simulink model "busdemo"  (Simulink 7.6)
settings: Solver=VariableStepDiscrete  StartTime=0.0  StopTime=10  MaxStep=.05  RelTol=1e-3
libraries: simulink x2
Description:
  | Demonstration model for vector, matrix, and composite signals
  | 
  | This model introduces you to the following Simulink(R) concepts:
  | 
  |  * Distinguishing vector, matrix, and bus/composite signals
  |  * Understanding signal line formats
  |  * Displaying and understanding signal dimensions
  |  * Using the Bus Creator and the Bus Selector blocks
  |  * Viewing matrix signals on a Simulink Scope
  |  * Highlighting blocks in the Simulink diagram
settings Model: Creator=The MathWorks Inc.  CovMetricSettings=d  ExtModeTrigMode=oneshot  ExtModeArmWhenConnect=off  ExtModeAutoUpdateStatusClock=off
settings DataIOCC: LimitDataPoints=off  SaveOutput=off  SignalLogging=off  SaveTime=off
settings OptimizationCC: BlockReduction=off  BooleanDataType=off  InlineInvariantSignals=on  InitFltsAndDblsToZero=on  BufferReusableBoundary=off
settings DebuggingCC: SaveWithParameterizedLinksMsg=none  SignalResolutionControl=TryResolveAllWithWarning  SolverPrmCheckMsg=none  MultiTaskDSMMsg=warning  MultiTaskCondExecSysMsg=none  IntegerOverflowMsg=none  BusObjectLabelMismatch=none
settings HardwareCC: TargetUnknown=on
settings RTWCC: IncludeERTFirstTime=on
settings GRTTargetCC: TargetFcnLib=ansi_tfl_tmw.mat

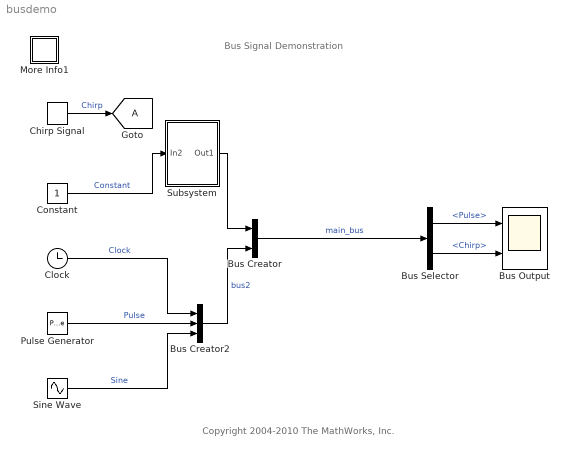
== system busdemo ==
  note: Bus Signal Demonstration
  note: Copyright 2004-2010 The MathWorks, Inc.
  Bus Creator : BusCreator  Inputs=2
  Bus Creator2 : BusCreator  Inputs=3
  Bus Selector : BusSelector  OutputSignals=bus2.Pulse,bus1.Chirp
  Bus Output : Scope  NumInputPorts=2
      settings: StartFcn=open_system(gcbh)  TimeRange=10  YMin=-3~-5  YMax=3~5  DataFormat=Structure
  Chirp Signal : simulink/Sources/Chirp Signal  SystemSampleTime=-1  f1=0.1  T=10  f2=5
  Clock : Clock
      settings: Decimation=10
  Constant : Constant
  More Info1 : Subsystem
      settings: OpenFcn=showdemo(bdroot(gcs))
      mask Display: disp('?')
  Pulse Generator : DiscretePulseGenerator
  Sine Wave : Sin  SampleTime=0
  Subsystem : Subsystem
  tag scope: A=global
  wires:
  Clock/1 -> Bus Creator2/1  "Clock"
  Pulse Generator/1 -> Bus Creator2/2  "Pulse"
  Sine Wave/1 -> Bus Creator2/3  "Sine"
  Constant/1 -> Subsystem/1(In2)  "Constant"
  Bus Creator/1 -> Bus Selector/1  "main_bus"
  Bus Selector/1 -> Bus Output/1  "<Pulse>"
  Bus Selector/2 -> Bus Output/2  "<Chirp>"
  Subsystem/1(Out1) -> Bus Creator/1
  Bus Creator2/1 -> Bus Creator/2  "bus2"
  Chirp Signal/1 -> [A]  "Chirp"

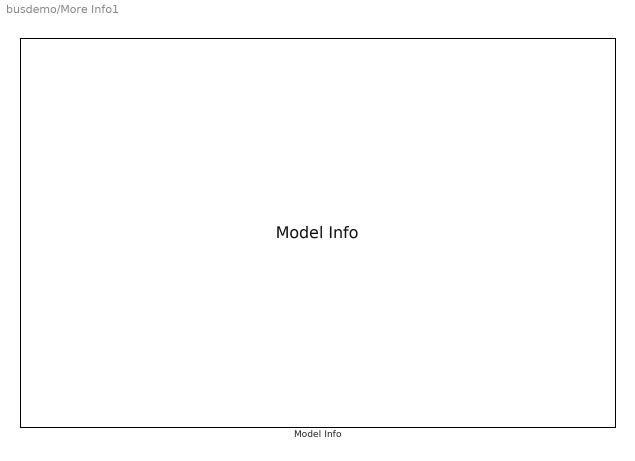
== system busdemo/More Info1 ==
  Model Info : simulink/Model-Wide Utilities/Model Info  InitialBlockCM=none  BlockCM=None  Frame=on  HorizontalTextAlignment=Left  LeftAlignmentValue=0.02  SourceBlockDiagram=busdemo  TagMaxNumber=20

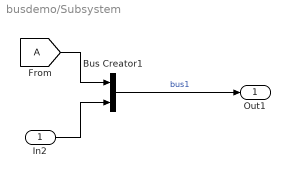
== system busdemo/Subsystem ==
  In2 : Inport
  Bus Creator1 : BusCreator  Inputs=2
  Out1 : Outport
  wires:
  [A] -> Bus Creator1/1
  Bus Creator1/1 -> Out1/1  "bus1"
  In2/1 -> Bus Creator1/2
